simulink model "step_input_sec_ord"  (R2024b)
settings: Solver=VariableStepAuto  StartTime=0.0  StopTime=10.0  RelTol=1e-3
settings Model: Creator=darkk157night  LastModifiedBy=darkk157night

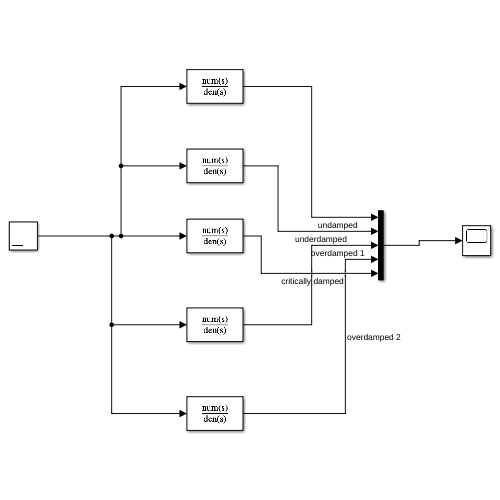
[thumbnail: Simulink's stored preview of the top-level diagram]
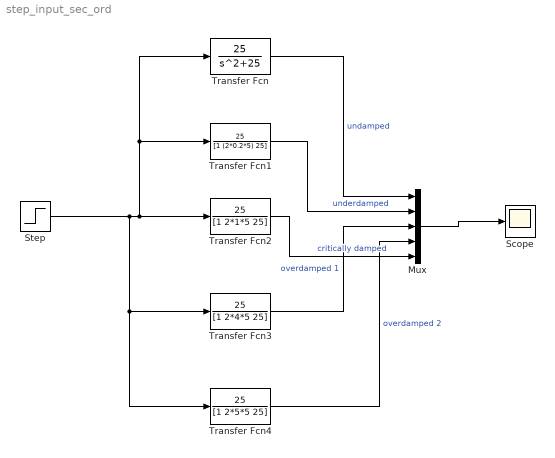
== system step_input_sec_ord ==
  Mux : Mux  Inputs=5
  Scope : Scope
  Step : Step  SampleTime=0
  Transfer Fcn : TransferFcn  Numerator=[25]  Denominator=[1 0 25]
  Transfer Fcn1 : TransferFcn  Numerator=[25]  Denominator=[1 (2*0.2*5) 25]
  Transfer Fcn2 : TransferFcn  Numerator=[25]  Denominator=[1 2*1*5 25]
  Transfer Fcn3 : TransferFcn  Numerator=[25]  Denominator=[1 2*4*5 25]
  Transfer Fcn4 : TransferFcn  Numerator=[25]  Denominator=[1 2*5*5 25]
  wires:
  Step/1 -> Transfer Fcn/1, Transfer Fcn1/1, Transfer Fcn2/1, Transfer Fcn4/1, Transfer Fcn3/1
  Transfer Fcn/1 -> Mux/1  "undamped"
  Transfer Fcn1/1 -> Mux/2  "underdamped"
  Transfer Fcn3/1 -> Mux/3  "overdamped 1"
  Transfer Fcn4/1 -> Mux/4  "overdamped 2"
  Mux/1 -> Scope/1
  Transfer Fcn2/1 -> Mux/5  "critically damped"
